simulink model "Lab_3_sim"  (R2021b)
settings: Solver=VariableStepAuto  StartTime=0.0  StopTime=czas_symulacji  RelTol=1e-3
values from neighbouring files (symbols this model uses):
  a0 = 5    [Lab_3.m]
  a1 = 6    [Lab_3.m]
  b = 4    [Lab_3.m]
  du = 1    [Lab_3.m]
  t0 = 10    [Lab_3.m]
  u0 = 3    [Lab_3.m]
  x0 = (b*u0)/a0    (= 2.4)    [Lab_3.m]
settings Model: Creator=Ovocsiak  LastModifiedBy=Ovocsiak
settings DataIOCC: ReturnWorkspaceOutputs=off

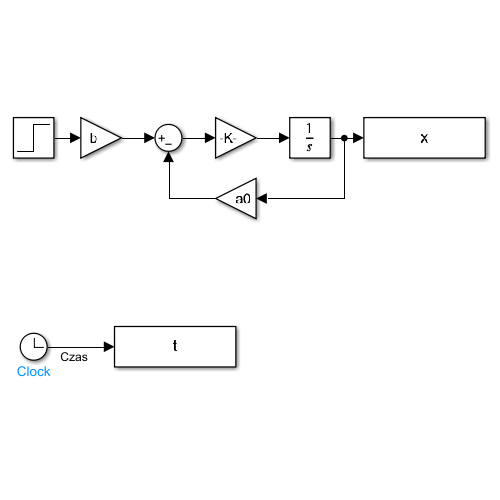
[thumbnail: Simulink's stored preview of the top-level diagram]
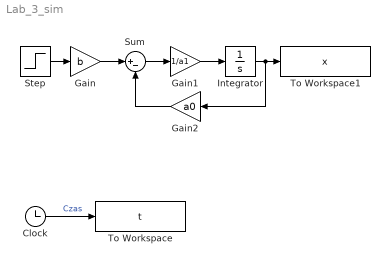
== system Lab_3_sim ==
  Clock : Clock
  Gain : Gain  Gain=b
  Gain1 : Gain  Gain=1/a1
  Gain2 : Gain  Gain=a0
  Integrator : Integrator  InitialCondition=x0
  Step : Step  Time=t0  Before=u0  After=u0 + du  SampleTime=0
  Sum : Sum  Inputs=|+-
  To Workspace : ToWorkspace  VariableName=t  SampleTime=-1
  To Workspace1 : ToWorkspace  VariableName=x  SampleTime=-1
  wires:
  Clock/1 -> To Workspace/1  "Czas"
  Step/1 -> Gain/1
  Gain/1 -> Sum/1
  Integrator/1 -> Gain2/1, To Workspace1/1
  Sum/1 -> Gain1/1
  Gain1/1 -> Integrator/1
  Gain2/1 -> Sum/2
